simulink model "Demo_V2X_RoadWorks_cs"  (R2014b)
settings: Solver=ode5  SolverMode=SingleTasking  StartTime=0.0  StopTime=18  FixedStep=1/100  RelTol=1e-3
PreLoadFcn:
  | mbxruntime.callbacks.PreLoadFcn(bdroot);
  | check_NUTS_defined;
  | 
  | assignin('base',['model_closed_' bdroot],false);
PostLoadFcn:
  | mbxruntime.callbacks.PostLoadFcn(bdroot);
InitFcn:
  | mbxruntime.callbacks.InitFcn(bdroot);
StartFcn:
  | mbxruntime.callbacks.StartFcn(bdroot);
StopFcn:
  | mbxruntime.callbacks.StopFcn(bdroot);
model workspace: external: MAT-File .\Demo_V2X_RoadWorks_cs_hws.mat (data not in the file)
undefined symbols (not defined in the file or in its folder): InitializeBus, mbxruntime, Newton, Raphson, tabledata
undefined symbols (not defined in the file): Demo_V2X_RoadWorks_cs_002408181c311178, Demo_V2X_RoadWorks_cs_02afd40c5576fd79, Demo_V2X_RoadWorks_cs_09062d95c4976b80, Demo_V2X_RoadWorks_cs_0ad60e46608f1bfe, Demo_V2X_RoadWorks_cs_0b386a01b2cd5e8d, Demo_V2X_RoadWorks_cs_0d795afaa024d2ee, Demo_V2X_RoadWorks_cs_104085e65c337077, Demo_V2X_RoadWorks_cs_126564f7b2997a49, Demo_V2X_RoadWorks_cs_15e6e2595e8bf329, Demo_V2X_RoadWorks_cs_16adfea7655bce18, Demo_V2X_RoadWorks_cs_18ab2686f8449f50, Demo_V2X_RoadWorks_cs_1c28437def32f9f6, Demo_V2X_RoadWorks_cs_1d541c73c3d8f25b, Demo_V2X_RoadWorks_cs_1fb1f994fe012d27, Demo_V2X_RoadWorks_cs_20c117b9827230b9, Demo_V2X_RoadWorks_cs_220b1226a84e3b37, Demo_V2X_RoadWorks_cs_24814049c8ab2e18, Demo_V2X_RoadWorks_cs_24a281220a6492a7, Demo_V2X_RoadWorks_cs_279aea126b4236ad, Demo_V2X_RoadWorks_cs_28eadd0b23e572db, Demo_V2X_RoadWorks_cs_291fe7210f9ba434, Demo_V2X_RoadWorks_cs_2fd90504f8814746, Demo_V2X_RoadWorks_cs_33c1737bfc1c651f, Demo_V2X_RoadWorks_cs_388e22d5b1056b8f, Demo_V2X_RoadWorks_cs_3e3a415e868663e7, Demo_V2X_RoadWorks_cs_45759eb0c1816b1e, Demo_V2X_RoadWorks_cs_45f301cf6c396570, Demo_V2X_RoadWorks_cs_47686124f5151dea, Demo_V2X_RoadWorks_cs_487931e8a8cef1d6, Demo_V2X_RoadWorks_cs_54cb5626dca53ab7, Demo_V2X_RoadWorks_cs_56c0a253fe7e7ec0, Demo_V2X_RoadWorks_cs_5921488c0ba4168e, Demo_V2X_RoadWorks_cs_5ca0c70551eea1b3, Demo_V2X_RoadWorks_cs_5cc6ddb60eb17926, Demo_V2X_RoadWorks_cs_5dda33a127b53dd9, Demo_V2X_RoadWorks_cs_60729aca19e3b8ea, Demo_V2X_RoadWorks_cs_61616eaaf58ec115, Demo_V2X_RoadWorks_cs_63af626c9fae5224, Demo_V2X_RoadWorks_cs_649c6af7b111a61f, Demo_V2X_RoadWorks_cs_64e2df335ac415c1, Demo_V2X_RoadWorks_cs_6530f1ae727e39fe, Demo_V2X_RoadWorks_cs_6837be8d052ff1e3, Demo_V2X_RoadWorks_cs_6e8b51a123f1a201, Demo_V2X_RoadWorks_cs_6f4ec518a68cacb3, Demo_V2X_RoadWorks_cs_74dac4a6b9859226, Demo_V2X_RoadWorks_cs_75671d8cae67d5b6, Demo_V2X_RoadWorks_cs_756d40a88ae84d39, Demo_V2X_RoadWorks_cs_77c7cbc4fa1cdaa5, Demo_V2X_RoadWorks_cs_7b9fbc44403bb8f3, Demo_V2X_RoadWorks_cs_7c118b74c8d14c00, Demo_V2X_RoadWorks_cs_7c4a172761f05beb, Demo_V2X_RoadWorks_cs_80b7a78efe24d5f1, Demo_V2X_RoadWorks_cs_82d65efce1f7c4ea, Demo_V2X_RoadWorks_cs_8be5dc2565229ce9, Demo_V2X_RoadWorks_cs_8dc36f0ab6cec640, Demo_V2X_RoadWorks_cs_91305dd1362bb00d, Demo_V2X_RoadWorks_cs_929c2ffed1faf33f, Demo_V2X_RoadWorks_cs_95615bcbc0d062f1, Demo_V2X_RoadWorks_cs_99a6391a40f894df, Demo_V2X_RoadWorks_cs_9caa19175765ea5d ... (+52)
libraries: PreScanSimulinkLibrary x34, simulink_extras x15, simulink x6
(part 16 of 16)

== matlab function Demo_V2X_RoadWorks_cs/Actros_2541_1/V2X_6201_DENM_Create ==
  data: PRESCAN_V2X_FIXED_DENM_MESSAGE_zero_init parameter Bus: PRESCAN_V2X_FIXED_DENM_MESSAGE; message output Bus: PRESCAN_V2X_FIXED_DENM_MESSAGE; z input
function message = update(PRESCAN_V2X_FIXED_DENM_MESSAGE_zero_init, z)
%#codegen

message = PRESCAN_V2X_FIXED_DENM_MESSAGE_zero_init;
message.HEADER.valid = true;

% The lines below are example assignments that can be uncommented
% and changed as needed to construct a message to be sent.

% message.DATA.header.protocolVersion = int32(1);
% message.DATA.header.messageID = int32(1);
% message.DATA.header.stationID = int32(1);
% message.DATA.denm.management.actionID.originatingStationID = int32(1);
% message.DATA.denm.management.actionID.sequenceNumber = int32(1);
% message.DATA.denm.management.eventPosition.positionConfidenceEllipse.semiMajorConfidence = int32(1);
% message.DATA.denm.management.eventPosition.positionConfidenceEllipse.semiMinorConfidence = int32(1);
% message.DATA.denm.management.eventPosition.positionConfidenceEllipse.semiMajorOrientation = int32(1);
% message.DATA.denm.management.eventPosition.altitude.altitudeValue = int32(1);
% message.DATA.denm.management.eventPosition.altitude.altitudeConfidence = int32(1);
% message.DATA.denm.management.eventPosition.latitude = int32(1);
% message.DATA.denm.management.eventPosition.longitude = int32(1);
% message.DATA.denm.management.detectionTime = int32(1);
% message.DATA.denm.management.referenceTime = int32(1);
% message.DATA.denm.management.termination = int32(1);
% message.DATA.denm.management.relevanceDistance = int32(1);
% message.DATA.denm.management.relevanceTrafficDirection = int32(1);
% message.DATA.denm.management.validityDuration = int32(1);
% message.DATA.denm.management.transmissionInterval = int32(1);
% message.DATA.denm.management.stationType = int32(1);
% message.DATA.denm.situation.eventType.causeCode = int32(1);
% message.DATA.denm.situation.eventType.subCauseCode = int32(1);
% message.DATA.denm.situation.linkedCause.causeCode = int32(1);
% message.DATA.denm.situation.linkedCause.subCauseCode = int32(1);
% message.DATA.denm.situation.eventHistory(1).eventPosition.deltaLatitude = int32(1);
% message.DATA.denm.situation.eventHistory(1).eventPosition.deltaLongitude = int32(1);
% message.DATA.denm.situation.eventHistory(1).eventPosition.deltaAltitude = int32(1);
% message.DATA.denm.situation.eventHistory(1).eventDeltaTime = int32(1);
% message.DATA.denm.situation.eventHistory(1).informationQuality = int32(1);
% message.DATA.denm.situation.informationQuality = int32(1);
% % message.DATA.denm.situation.eventHistory(1) is an array
% message.DATA.denm.location.eventSpeed.speedValue = int32(1);
% message.DATA.denm.location.eventSpeed.speedConfidence = int32(1);
% message.DATA.denm.location.eventPositionHeading.headingValue = int32(1);
% message.DATA.denm.location.eventPositionHeading.headingConfidence = int32(1);
% message.DATA.denm.location.traces(1).pathPosition.deltaLatitude = int32(1);
% message.DATA.denm.location.traces(1).pathPosition.deltaLongitude = int32(1);
% message.DATA.denm.location.traces(1).pathPosition.deltaAltitude = int32(1);
% message.DATA.denm.location.traces(1).pathDeltaTime = int32(1);
% % message.DATA.denm.location.traces(1) is an array
% message.DATA.denm.location.roadType = int32(1);
% message.DATA.denm.alacarte.impactReduction.heightLonCarrLeft = int32(1);
% message.DATA.denm.alacarte.impactReduction.heightLonCarrRight = int32(1);
% message.DATA.denm.alacarte.impactReduction.posLonCarrLeft = int32(1);
% message.DATA.denm.alacarte.impactReduction.posLonCarrRight = int32(1);
% % message.DATA.denm.alacarte.impactReduction.positionOfPillars(1) is an array
% message.DATA.denm.alacarte.impactReduction.posCentMass = int32(1);
% message.DATA.denm.alacarte.impactReduction.wheelBaseVehicle = int32(1);
% message.DATA.denm.alacarte.impactReduction.turningRadius = int32(1);
% message.DATA.denm.alacarte.impactReduction.posFrontAx = int32(1);
% message.DATA.denm.alacarte.impactReduction.positionOfOccupants = int32(1);
% message.DATA.denm.alacarte.impactReduction.vehicleMass = int32(1);
% message.DATA.denm.alacarte.impactReduction.requestResponseIndication = int32(1);
% message.DATA.denm.alacarte.roadWorks.closedLanes.hardShoulderStatus = int32(1);
% message.DATA.denm.alacarte.roadWorks.closedLanes.drivingLaneStatus = int32(1);
% message.DATA.denm.alacarte.roadWorks.incidentIndication.causeCode = int32(1);
% message.DATA.denm.alacarte.roadWorks.incidentIndication.subCauseCode = int32(1);
% message.DATA.denm.alacarte.roadWorks.recommendedPath(1).positionConfidenceEllipse.semiMajorConfidence = int32(1);
% message.DATA.denm.alacarte.roadWorks.recommendedPath(1).positionConfidenceEllipse.semiMinorConfidence = int32(1);
% message.DATA.denm.alacarte.roadWorks.recommendedPath(1).positionConfidenceEllipse.semiMajorOrientation = int32(1);
% message.DATA.denm.alacarte.roadWorks.recommendedPath(1).altitude.altitudeValue = int32(1);
% message.DATA.denm.alacarte.roadWorks.recommendedPath(1).altitude.altitudeConfidence = int32(1);
% message.DATA.denm.alacarte.roadWorks.recommendedPath(1).latitude = int32(1);
% message.DATA.denm.alacarte.roadWorks.recommendedPath(1).longitude = int32(1);
% message.DATA.denm.alacarte.roadWorks.startingPointSpeedLimit.deltaLatitude = int32(1);
% message.DATA.denm.alacarte.roadWorks.startingPointSpeedLimit.deltaLongitude = int32(1);
% message.DATA.denm.alacarte.roadWorks.startingPointSpeedLimit.deltaAltitude = int32(1);
% message.DATA.denm.alacarte.roadWorks.referenceDenms(1).originatingStationID = int32(1);
% message.DATA.denm.alacarte.roadWorks.referenceDenms(1).sequenceNumber = int32(1);
% message.DATA.denm.alacarte.roadWorks.lightBarSirenInUse = int32(1);
% % message.DATA.denm.alacarte.roadWorks.restriction(1) is an array
% message.DATA.denm.alacarte.roadWorks.speedLimit = int32(1);
% % message.DATA.denm.alacarte.roadWorks.recommendedPath(1) is an array
% message.DATA.denm.alacarte.roadWorks.trafficFlowRule = int32(1);
% % message.DATA.denm.alacarte.roadWorks.referenceDenms(1) is an array
% message.DATA.denm.alacarte.stationaryVehicle.stationaryCause.causeCode = int32(1);
% message.DATA.denm.alacarte.stationaryVehicle.stationaryCause.subCauseCode = int32(1);
% message.DATA.denm.alacarte.stationaryVehicle.carryingDangerousGoods.dangerousGoodsType = int32(1);
% message.DATA.denm.alacarte.stationaryVehicle.carryingDangerousGoods.unNumber = int32(1);
% message.DATA.denm.alacarte.stationaryVehicle.carryingDangerousGoods.elevatedTemperature = logical(1);
% message.DATA.denm.alacarte.stationaryVehicle.carryingDangerousGoods.tunnelsRestricted = logical(1);
% message.DATA.denm.alacarte.stationaryVehicle.carryingDangerousGoods.limitedQuantity = logical(1);
% message.DATA.denm.alacarte.stationaryVehicle.carryingDangerousGoods.emergencyActionCode = int8(zeros(24, 1)); % Array up to 24 bytes
% message.DATA.denm.alacarte.stationaryVehicle.carryingDangerousGoods.phoneNumber = int8(zeros(24, 1)); % Array up to 24 bytes
% message.DATA.denm.alacarte.stationaryVehicle.carryingDangerousGoods.companyName = int8(zeros(24, 1)); % Array up to 24 bytes
% message.DATA.denm.alacarte.stationaryVehicle.vehicleIdentification.wMInumber = int8(zeros(3, 1)); % Array up to 3 bytes
% message.DATA.denm.alacarte.stationaryVehicle.vehicleIdentification.vDS = int8(zeros(6, 1)); % Array up to 6 bytes
% message.DATA.denm.alacarte.stationaryVehicle.stationarySince = int32(1);
% message.DATA.denm.alacarte.stationaryVehicle.numberOfOccupants = int32(1);
% message.DATA.denm.alacarte.stationaryVehicle.energyStorageType = int32(1);
% message.DATA.denm.alacarte.lanePosition = int32(1);
% message.DATA.denm.alacarte.externalTemperature = int32(1);
% message.DATA.denm.alacarte.positioningSolution = int32(1);

== matlab function Demo_V2X_RoadWorks_cs/Actros_1860_1/V2X_6202_CAM_Create ==
  data: PRESCAN_V2X_FIXED_CAM_MESSAGE_zero_init parameter Bus: PRESCAN_V2X_FIXED_CAM_MESSAGE; message output Bus: PRESCAN_V2X_FIXED_CAM_MESSAGE; z input
function message = update(PRESCAN_V2X_FIXED_CAM_MESSAGE_zero_init, z)
%#codegen

message = PRESCAN_V2X_FIXED_CAM_MESSAGE_zero_init;
message.HEADER.valid = true;

% The lines below are example assignments that can be uncommented
% and changed as needed to construct a message to be sent.

% message.DATA.header.protocolVersion = int32(1);
% message.DATA.header.messageID = int32(1);
% message.DATA.header.stationID = int32(1);
% message.DATA.cam.camParameters.basicContainer.referencePosition.positionConfidenceEllipse.semiMajorConfidence = int32(1);
% message.DATA.cam.camParameters.basicContainer.referencePosition.positionConfidenceEllipse.semiMinorConfidence = int32(1);
% message.DATA.cam.camParameters.basicContainer.referencePosition.positionConfidenceEllipse.semiMajorOrientation = int32(1);
% message.DATA.cam.camParameters.basicContainer.referencePosition.altitude.altitudeValue = int32(1);
% message.DATA.cam.camParameters.basicContainer.referencePosition.altitude.altitudeConfidence = int32(1);
% message.DATA.cam.camParameters.basicContainer.referencePosition.latitude = int32(1);
% message.DATA.cam.camParameters.basicContainer.referencePosition.longitude = int32(1);
% message.DATA.cam.camParameters.basicContainer.stationType = int32(1);
% message.DATA.cam.camParameters.highFrequencyContainer.basicVehicleContainerHighFrequency.heading.headingValue = int32(1);
% message.DATA.cam.camParameters.highFrequencyContainer.basicVehicleContainerHighFrequency.heading.headingConfidence = int32(1);
% message.DATA.cam.camParameters.highFrequencyContainer.basicVehicleContainerHighFrequency.speed.speedValue = int32(1);
% message.DATA.cam.camParameters.highFrequencyContainer.basicVehicleContainerHighFrequency.speed.speedConfidence = int32(1);
% message.DATA.cam.camParameters.highFrequencyContainer.basicVehicleContainerHighFrequency.vehicleLength.vehicleLengthValue = int32(1);
% message.DATA.cam.camParameters.highFrequencyContainer.basicVehicleContainerHighFrequency.vehicleLength.vehicleLengthConfidenceIndication = int32(1);
% message.DATA.cam.camParameters.highFrequencyContainer.basicVehicleContainerHighFrequency.longitudinalAcceleration.longitudinalAccelerationValue = int32(1);
% message.DATA.cam.camParameters.highFrequencyContainer.basicVehicleContainerHighFrequency.longitudinalAcceleration.longitudinalAccelerationConfidence = int32(1);
% message.DATA.cam.camParameters.highFrequencyContainer.basicVehicleContainerHighFrequency.curvature.curvatureValue = int32(1);
% message.DATA.cam.camParameters.highFrequencyContainer.basicVehicleContainerHighFrequency.curvature.curvatureConfidence = int32(1);
% message.DATA.cam.camParameters.highFrequencyContainer.basicVehicleContainerHighFrequency.yawRate.yawRateValue = int32(1);
% message.DATA.cam.camParameters.highFrequencyContainer.basicVehicleContainerHighFrequency.yawRate.yawRateConfidence = int32(1);
% message.DATA.cam.camParameters.highFrequencyContainer.basicVehicleContainerHighFrequency.steeringWheelAngle.steeringWheelAngleValue = int32(1);
% message.DATA.cam.camParameters.highFrequencyContainer.basicVehicleContainerHighFrequency.steeringWheelAngle.steeringWheelAngleConfidence = int32(1);
% message.DATA.cam.camParameters.highFrequencyContainer.basicVehicleContainerHighFrequency.lateralAcceleration.lateralAccelerationValue = int32(1);
% message.DATA.cam.camParameters.highFrequencyContainer.basicVehicleContainerHighFrequency.lateralAcceleration.lateralAccelerationConfidence = int32(1);
% message.DATA.cam.camParameters.highFrequencyContainer.basicVehicleContainerHighFrequency.verticalAcceleration.verticalAccelerationValue = int32(1);
% message.DATA.cam.camParameters.highFrequencyContainer.basicVehicleContainerHighFrequency.verticalAcceleration.verticalAccelerationConfidence = int32(1);
% message.DATA.cam.camParameters.highFrequencyContainer.basicVehicleContainerHighFrequency.cenDsrcTollingZone.protectedZoneLatitude = int32(1);
% message.DATA.cam.camParameters.highFrequencyContainer.basicVehicleContainerHighFrequency.cenDsrcTollingZone.protectedZoneLongitude = int32(1);
% message.DATA.cam.camParameters.highFrequencyContainer.basicVehicleContainerHighFrequency.cenDsrcTollingZone.cenDsrcTollingZoneID = int32(1);
% message.DATA.cam.camParameters.highFrequencyContainer.basicVehicleContainerHighFrequency.driveDirection = int32(1);
% message.DATA.cam.camParameters.highFrequencyContainer.basicVehicleContainerHighFrequency.vehicleWidth = int32(1);
% message.DATA.cam.camParameters.highFrequencyContainer.basicVehicleContainerHighFrequency.curvatureCalculationMode = int32(1);
% message.DATA.cam.camParameters.highFrequencyContainer.basicVehicleContainerHighFrequency.accelerationControl = int32(1);
% message.DATA.cam.camParameters.highFrequencyContainer.basicVehicleContainerHighFrequency.lanePosition = int32(1);
% message.DATA.cam.camParameters.highFrequencyContainer.basicVehicleContainerHighFrequency.performanceClass = int32(1);
% message.DATA.cam.camParameters.highFrequencyContainer.rsuContainerHighFrequency.protectedCommunicationZonesRSU(1).protectedZoneType = int32(1);
% message.DATA.cam.camParameters.highFrequencyContainer.rsuContainerHighFrequency.protectedCommunicationZonesRSU(1).expiryTime = int32(1);
% message.DATA.cam.camParameters.highFrequencyContainer.rsuContainerHighFrequency.protectedCommunicationZonesRSU(1).protectedZoneLatitude = int32(1);
% message.DATA.cam.camParameters.highFrequencyContainer.rsuContainerHighFrequency.protectedCommunicationZonesRSU(1).protectedZoneLongitude = int32(1);
% message.DATA.cam.camParameters.highFrequencyContainer.rsuContainerHighFrequency.protectedCommunicationZonesRSU(1).protectedZoneRadius = int32(1);
% message.DATA.cam.camParameters.highFrequencyContainer.rsuContainerHighFrequency.protectedCommunicationZonesRSU(1).protectedZoneID = int32(1);
% % message.DATA.cam.camParameters.highFrequencyContainer.rsuContainerHighFrequency.protectedCommunicationZonesRSU(1) is an array
% message.DATA.cam.camParameters.lowFrequencyContainer.basicVehicleContainerLowFrequency.pathHistory(1).pathPosition.deltaLatitude = int32(1);
% message.DATA.cam.camParameters.lowFrequencyContainer.basicVehicleContainerLowFrequency.pathHistory(1).pathPosition.deltaLongitude = int32(1);
% message.DATA.cam.camParameters.lowFrequencyContainer.basicVehicleContainerLowFrequency.pathHistory(1).pathPosition.deltaAltitude = int32(1);
% message.DATA.cam.camParameters.lowFrequencyContainer.basicVehicleContainerLowFrequency.pathHistory(1).pathDeltaTime = int32(1);
% message.DATA.cam.camParameters.lowFrequencyContainer.basicVehicleContainerLowFrequency.vehicleRole = int32(1);
% message.DATA.cam.camParameters.lowFrequencyContainer.basicVehicleContainerLowFrequency.exteriorLights = int32(1);
% % message.DATA.cam.camParameters.lowFrequencyContainer.basicVehicleContainerLowFrequency.pathHistory(1) is an array
% message.DATA.cam.camParameters.specialVehicleContainer.publicTransportContainer.ptActivation.ptActivationType = int32(1);
% message.DATA.cam.camParameters.specialVehicleContainer.publicTransportContainer.ptActivation.ptActivationData = int8(zeros(20, 1)); % Array up to 20 bytes
% message.DATA.cam.camParameters.specialVehicleContainer.publicTransportContainer.embarkationStatus = logical(1);
% message.DATA.cam.camParameters.specialVehicleContainer.specialTransportContainer.specialTransportType = int32(1);
% message.DATA.cam.camParameters.specialVehicleContainer.specialTransportContainer.lightBarSirenInUse = int32(1);
% message.DATA.cam.camParameters.specialVehicleContainer.dangerousGoodsContainer.dangerousGoodsBasic = int32(1);
% message.DATA.cam.camParameters.specialVehicleContainer.roadWorksContainerBasic.closedLanes.hardShoulderStatus = int32(1);
% message.DATA.cam.camParameters.specialVehicleContainer.roadWorksContainerBasic.closedLanes.drivingLaneStatus = int32(1);
% message.DATA.cam.camParameters.specialVehicleContainer.roadWorksContainerBasic.roadworksSubCauseCode = int32(1);
% message.DATA.cam.camParameters.specialVehicleContainer.roadWorksContainerBasic.lightBarSirenInUse = int32(1);
% message.DATA.cam.camParameters.specialVehicleContainer.rescueContainer.lightBarSirenInUse = int32(1);
% message.DATA.cam.camParameters.specialVehicleContainer.emergencyContainer.incidentIndication.causeCode = int32(1);
% message.DATA.cam.camParameters.specialVehicleContainer.emergencyContainer.incidentIndication.subCauseCode = int32(1);
% message.DATA.cam.camParameters.specialVehicleContainer.emergencyContainer.lightBarSirenInUse = int32(1);
% message.DATA.cam.camParameters.specialVehicleContainer.emergencyContainer.emergencyPriority = int32(1);
% message.DATA.cam.camParameters.specialVehicleContainer.safetyCarContainer.incidentIndication.causeCode = int32(1);
% message.DATA.cam.camParameters.specialVehicleContainer.safetyCarContainer.incidentIndication.subCauseCode = int32(1);
% message.DATA.cam.camParameters.specialVehicleContainer.safetyCarContainer.lightBarSirenInUse = int32(1);
% message.DATA.cam.camParameters.specialVehicleContainer.safetyCarContainer.trafficRule = int32(1);
% message.DATA.cam.camParameters.specialVehicleContainer.safetyCarContainer.speedLimit = int32(1);
% message.DATA.cam.generationDeltaTime = int32(1);

== matlab function Demo_V2X_RoadWorks_cs/Actros_1860_1/V2X_6202_DENM_Create ==
  data: PRESCAN_V2X_FIXED_DENM_MESSAGE_zero_init parameter Bus: PRESCAN_V2X_FIXED_DENM_MESSAGE; message output Bus: PRESCAN_V2X_FIXED_DENM_MESSAGE; z input
function message = update(PRESCAN_V2X_FIXED_DENM_MESSAGE_zero_init, z)
%#codegen

message = PRESCAN_V2X_FIXED_DENM_MESSAGE_zero_init;
message.HEADER.valid = true;

% The lines below are example assignments that can be uncommented
% and changed as needed to construct a message to be sent.

% message.DATA.header.protocolVersion = int32(1);
% message.DATA.header.messageID = int32(1);
% message.DATA.header.stationID = int32(1);
% message.DATA.denm.management.actionID.originatingStationID = int32(1);
% message.DATA.denm.management.actionID.sequenceNumber = int32(1);
% message.DATA.denm.management.eventPosition.positionConfidenceEllipse.semiMajorConfidence = int32(1);
% message.DATA.denm.management.eventPosition.positionConfidenceEllipse.semiMinorConfidence = int32(1);
% message.DATA.denm.management.eventPosition.positionConfidenceEllipse.semiMajorOrientation = int32(1);
% message.DATA.denm.management.eventPosition.altitude.altitudeValue = int32(1);
% message.DATA.denm.management.eventPosition.altitude.altitudeConfidence = int32(1);
% message.DATA.denm.management.eventPosition.latitude = int32(1);
% message.DATA.denm.management.eventPosition.longitude = int32(1);
% message.DATA.denm.management.detectionTime = int32(1);
% message.DATA.denm.management.referenceTime = int32(1);
% message.DATA.denm.management.termination = int32(1);
% message.DATA.denm.management.relevanceDistance = int32(1);
% message.DATA.denm.management.relevanceTrafficDirection = int32(1);
% message.DATA.denm.management.validityDuration = int32(1);
% message.DATA.denm.management.transmissionInterval = int32(1);
% message.DATA.denm.management.stationType = int32(1);
% message.DATA.denm.situation.eventType.causeCode = int32(1);
% message.DATA.denm.situation.eventType.subCauseCode = int32(1);
% message.DATA.denm.situation.linkedCause.causeCode = int32(1);
% message.DATA.denm.situation.linkedCause.subCauseCode = int32(1);
% message.DATA.denm.situation.eventHistory(1).eventPosition.deltaLatitude = int32(1);
% message.DATA.denm.situation.eventHistory(1).eventPosition.deltaLongitude = int32(1);
% message.DATA.denm.situation.eventHistory(1).eventPosition.deltaAltitude = int32(1);
% message.DATA.denm.situation.eventHistory(1).eventDeltaTime = int32(1);
% message.DATA.denm.situation.eventHistory(1).informationQuality = int32(1);
% message.DATA.denm.situation.informationQuality = int32(1);
% % message.DATA.denm.situation.eventHistory(1) is an array
% message.DATA.denm.location.eventSpeed.speedValue = int32(1);
% message.DATA.denm.location.eventSpeed.speedConfidence = int32(1);
% message.DATA.denm.location.eventPositionHeading.headingValue = int32(1);
% message.DATA.denm.location.eventPositionHeading.headingConfidence = int32(1);
% message.DATA.denm.location.traces(1).pathPosition.deltaLatitude = int32(1);
% message.DATA.denm.location.traces(1).pathPosition.deltaLongitude = int32(1);
% message.DATA.denm.location.traces(1).pathPosition.deltaAltitude = int32(1);
% message.DATA.denm.location.traces(1).pathDeltaTime = int32(1);
% % message.DATA.denm.location.traces(1) is an array
% message.DATA.denm.location.roadType = int32(1);
% message.DATA.denm.alacarte.impactReduction.heightLonCarrLeft = int32(1);
% message.DATA.denm.alacarte.impactReduction.heightLonCarrRight = int32(1);
% message.DATA.denm.alacarte.impactReduction.posLonCarrLeft = int32(1);
% message.DATA.denm.alacarte.impactReduction.posLonCarrRight = int32(1);
% % message.DATA.denm.alacarte.impactReduction.positionOfPillars(1) is an array
% message.DATA.denm.alacarte.impactReduction.posCentMass = int32(1);
% message.DATA.denm.alacarte.impactReduction.wheelBaseVehicle = int32(1);
% message.DATA.denm.alacarte.impactReduction.turningRadius = int32(1);
% message.DATA.denm.alacarte.impactReduction.posFrontAx = int32(1);
% message.DATA.denm.alacarte.impactReduction.positionOfOccupants = int32(1);
% message.DATA.denm.alacarte.impactReduction.vehicleMass = int32(1);
% message.DATA.denm.alacarte.impactReduction.requestResponseIndication = int32(1);
% message.DATA.denm.alacarte.roadWorks.closedLanes.hardShoulderStatus = int32(1);
% message.DATA.denm.alacarte.roadWorks.closedLanes.drivingLaneStatus = int32(1);
% message.DATA.denm.alacarte.roadWorks.incidentIndication.causeCode = int32(1);
% message.DATA.denm.alacarte.roadWorks.incidentIndication.subCauseCode = int32(1);
% message.DATA.denm.alacarte.roadWorks.recommendedPath(1).positionConfidenceEllipse.semiMajorConfidence = int32(1);
% message.DATA.denm.alacarte.roadWorks.recommendedPath(1).positionConfidenceEllipse.semiMinorConfidence = int32(1);
% message.DATA.denm.alacarte.roadWorks.recommendedPath(1).positionConfidenceEllipse.semiMajorOrientation = int32(1);
% message.DATA.denm.alacarte.roadWorks.recommendedPath(1).altitude.altitudeValue = int32(1);
% message.DATA.denm.alacarte.roadWorks.recommendedPath(1).altitude.altitudeConfidence = int32(1);
% message.DATA.denm.alacarte.roadWorks.recommendedPath(1).latitude = int32(1);
% message.DATA.denm.alacarte.roadWorks.recommendedPath(1).longitude = int32(1);
% message.DATA.denm.alacarte.roadWorks.startingPointSpeedLimit.deltaLatitude = int32(1);
% message.DATA.denm.alacarte.roadWorks.startingPointSpeedLimit.deltaLongitude = int32(1);
% message.DATA.denm.alacarte.roadWorks.startingPointSpeedLimit.deltaAltitude = int32(1);
% message.DATA.denm.alacarte.roadWorks.referenceDenms(1).originatingStationID = int32(1);
% message.DATA.denm.alacarte.roadWorks.referenceDenms(1).sequenceNumber = int32(1);
% message.DATA.denm.alacarte.roadWorks.lightBarSirenInUse = int32(1);
% % message.DATA.denm.alacarte.roadWorks.restriction(1) is an array
% message.DATA.denm.alacarte.roadWorks.speedLimit = int32(1);
% % message.DATA.denm.alacarte.roadWorks.recommendedPath(1) is an array
% message.DATA.denm.alacarte.roadWorks.trafficFlowRule = int32(1);
% % message.DATA.denm.alacarte.roadWorks.referenceDenms(1) is an array
% message.DATA.denm.alacarte.stationaryVehicle.stationaryCause.causeCode = int32(1);
% message.DATA.denm.alacarte.stationaryVehicle.stationaryCause.subCauseCode = int32(1);
% message.DATA.denm.alacarte.stationaryVehicle.carryingDangerousGoods.dangerousGoodsType = int32(1);
% message.DATA.denm.alacarte.stationaryVehicle.carryingDangerousGoods.unNumber = int32(1);
% message.DATA.denm.alacarte.stationaryVehicle.carryingDangerousGoods.elevatedTemperature = logical(1);
% message.DATA.denm.alacarte.stationaryVehicle.carryingDangerousGoods.tunnelsRestricted = logical(1);
% message.DATA.denm.alacarte.stationaryVehicle.carryingDangerousGoods.limitedQuantity = logical(1);
% message.DATA.denm.alacarte.stationaryVehicle.carryingDangerousGoods.emergencyActionCode = int8(zeros(24, 1)); % Array up to 24 bytes
% message.DATA.denm.alacarte.stationaryVehicle.carryingDangerousGoods.phoneNumber = int8(zeros(24, 1)); % Array up to 24 bytes
% message.DATA.denm.alacarte.stationaryVehicle.carryingDangerousGoods.companyName = int8(zeros(24, 1)); % Array up to 24 bytes
% message.DATA.denm.alacarte.stationaryVehicle.vehicleIdentification.wMInumber = int8(zeros(3, 1)); % Array up to 3 bytes
% message.DATA.denm.alacarte.stationaryVehicle.vehicleIdentification.vDS = int8(zeros(6, 1)); % Array up to 6 bytes
% message.DATA.denm.alacarte.stationaryVehicle.stationarySince = int32(1);
% message.DATA.denm.alacarte.stationaryVehicle.numberOfOccupants = int32(1);
% message.DATA.denm.alacarte.stationaryVehicle.energyStorageType = int32(1);
% message.DATA.denm.alacarte.lanePosition = int32(1);
% message.DATA.denm.alacarte.externalTemperature = int32(1);
% message.DATA.denm.alacarte.positioningSolution = int32(1);

== matlab function Demo_V2X_RoadWorks_cs/CarTrailer_SingleAxle_1/V2X_6114_CAM_Create ==
  data: PRESCAN_V2X_FIXED_CAM_MESSAGE_zero_init parameter Bus: PRESCAN_V2X_FIXED_CAM_MESSAGE; message output Bus: PRESCAN_V2X_FIXED_CAM_MESSAGE; z input
function message = update(PRESCAN_V2X_FIXED_CAM_MESSAGE_zero_init, z)
%#codegen

message = PRESCAN_V2X_FIXED_CAM_MESSAGE_zero_init;
message.HEADER.valid = true;

% The lines below are example assignments that can be uncommented
% and changed as needed to construct a message to be sent.

% message.DATA.header.protocolVersion = int32(1);
% message.DATA.header.messageID = int32(1);
% message.DATA.header.stationID = int32(1);
% message.DATA.cam.camParameters.basicContainer.referencePosition.positionConfidenceEllipse.semiMajorConfidence = int32(1);
% message.DATA.cam.camParameters.basicContainer.referencePosition.positionConfidenceEllipse.semiMinorConfidence = int32(1);
% message.DATA.cam.camParameters.basicContainer.referencePosition.positionConfidenceEllipse.semiMajorOrientation = int32(1);
% message.DATA.cam.camParameters.basicContainer.referencePosition.altitude.altitudeValue = int32(1);
% message.DATA.cam.camParameters.basicContainer.referencePosition.altitude.altitudeConfidence = int32(1);
% message.DATA.cam.camParameters.basicContainer.referencePosition.latitude = int32(1);
% message.DATA.cam.camParameters.basicContainer.referencePosition.longitude = int32(1);
% message.DATA.cam.camParameters.basicContainer.stationType = int32(1);
% message.DATA.cam.camParameters.highFrequencyContainer.basicVehicleContainerHighFrequency.heading.headingValue = int32(1);
% message.DATA.cam.camParameters.highFrequencyContainer.basicVehicleContainerHighFrequency.heading.headingConfidence = int32(1);
% message.DATA.cam.camParameters.highFrequencyContainer.basicVehicleContainerHighFrequency.speed.speedValue = int32(1);
% message.DATA.cam.camParameters.highFrequencyContainer.basicVehicleContainerHighFrequency.speed.speedConfidence = int32(1);
% message.DATA.cam.camParameters.highFrequencyContainer.basicVehicleContainerHighFrequency.vehicleLength.vehicleLengthValue = int32(1);
% message.DATA.cam.camParameters.highFrequencyContainer.basicVehicleContainerHighFrequency.vehicleLength.vehicleLengthConfidenceIndication = int32(1);
% message.DATA.cam.camParameters.highFrequencyContainer.basicVehicleContainerHighFrequency.longitudinalAcceleration.longitudinalAccelerationValue = int32(1);
% message.DATA.cam.camParameters.highFrequencyContainer.basicVehicleContainerHighFrequency.longitudinalAcceleration.longitudinalAccelerationConfidence = int32(1);
% message.DATA.cam.camParameters.highFrequencyContainer.basicVehicleContainerHighFrequency.curvature.curvatureValue = int32(1);
% message.DATA.cam.camParameters.highFrequencyContainer.basicVehicleContainerHighFrequency.curvature.curvatureConfidence = int32(1);
% message.DATA.cam.camParameters.highFrequencyContainer.basicVehicleContainerHighFrequency.yawRate.yawRateValue = int32(1);
% message.DATA.cam.camParameters.highFrequencyContainer.basicVehicleContainerHighFrequency.yawRate.yawRateConfidence = int32(1);
% message.DATA.cam.camParameters.highFrequencyContainer.basicVehicleContainerHighFrequency.steeringWheelAngle.steeringWheelAngleValue = int32(1);
% message.DATA.cam.camParameters.highFrequencyContainer.basicVehicleContainerHighFrequency.steeringWheelAngle.steeringWheelAngleConfidence = int32(1);
% message.DATA.cam.camParameters.highFrequencyContainer.basicVehicleContainerHighFrequency.lateralAcceleration.lateralAccelerationValue = int32(1);
% message.DATA.cam.camParameters.highFrequencyContainer.basicVehicleContainerHighFrequency.lateralAcceleration.lateralAccelerationConfidence = int32(1);
% message.DATA.cam.camParameters.highFrequencyContainer.basicVehicleContainerHighFrequency.verticalAcceleration.verticalAccelerationValue = int32(1);
% message.DATA.cam.camParameters.highFrequencyContainer.basicVehicleContainerHighFrequency.verticalAcceleration.verticalAccelerationConfidence = int32(1);
% message.DATA.cam.camParameters.highFrequencyContainer.basicVehicleContainerHighFrequency.cenDsrcTollingZone.protectedZoneLatitude = int32(1);
% message.DATA.cam.camParameters.highFrequencyContainer.basicVehicleContainerHighFrequency.cenDsrcTollingZone.protectedZoneLongitude = int32(1);
% message.DATA.cam.camParameters.highFrequencyContainer.basicVehicleContainerHighFrequency.cenDsrcTollingZone.cenDsrcTollingZoneID = int32(1);
% message.DATA.cam.camParameters.highFrequencyContainer.basicVehicleContainerHighFrequency.driveDirection = int32(1);
% message.DATA.cam.camParameters.highFrequencyContainer.basicVehicleContainerHighFrequency.vehicleWidth = int32(1);
% message.DATA.cam.camParameters.highFrequencyContainer.basicVehicleContainerHighFrequency.curvatureCalculationMode = int32(1);
% message.DATA.cam.camParameters.highFrequencyContainer.basicVehicleContainerHighFrequency.accelerationControl = int32(1);
% message.DATA.cam.camParameters.highFrequencyContainer.basicVehicleContainerHighFrequency.lanePosition = int32(1);
% message.DATA.cam.camParameters.highFrequencyContainer.basicVehicleContainerHighFrequency.performanceClass = int32(1);
% message.DATA.cam.camParameters.highFrequencyContainer.rsuContainerHighFrequency.protectedCommunicationZonesRSU(1).protectedZoneType = int32(1);
% message.DATA.cam.camParameters.highFrequencyContainer.rsuContainerHighFrequency.protectedCommunicationZonesRSU(1).expiryTime = int32(1);
% message.DATA.cam.camParameters.highFrequencyContainer.rsuContainerHighFrequency.protectedCommunicationZonesRSU(1).protectedZoneLatitude = int32(1);
% message.DATA.cam.camParameters.highFrequencyContainer.rsuContainerHighFrequency.protectedCommunicationZonesRSU(1).protectedZoneLongitude = int32(1);
% message.DATA.cam.camParameters.highFrequencyContainer.rsuContainerHighFrequency.protectedCommunicationZonesRSU(1).protectedZoneRadius = int32(1);
% message.DATA.cam.camParameters.highFrequencyContainer.rsuContainerHighFrequency.protectedCommunicationZonesRSU(1).protectedZoneID = int32(1);
% % message.DATA.cam.camParameters.highFrequencyContainer.rsuContainerHighFrequency.protectedCommunicationZonesRSU(1) is an array
% message.DATA.cam.camParameters.lowFrequencyContainer.basicVehicleContainerLowFrequency.pathHistory(1).pathPosition.deltaLatitude = int32(1);
% message.DATA.cam.camParameters.lowFrequencyContainer.basicVehicleContainerLowFrequency.pathHistory(1).pathPosition.deltaLongitude = int32(1);
% message.DATA.cam.camParameters.lowFrequencyContainer.basicVehicleContainerLowFrequency.pathHistory(1).pathPosition.deltaAltitude = int32(1);
% message.DATA.cam.camParameters.lowFrequencyContainer.basicVehicleContainerLowFrequency.pathHistory(1).pathDeltaTime = int32(1);
% message.DATA.cam.camParameters.lowFrequencyContainer.basicVehicleContainerLowFrequency.vehicleRole = int32(1);
% message.DATA.cam.camParameters.lowFrequencyContainer.basicVehicleContainerLowFrequency.exteriorLights = int32(1);
% % message.DATA.cam.camParameters.lowFrequencyContainer.basicVehicleContainerLowFrequency.pathHistory(1) is an array
% message.DATA.cam.camParameters.specialVehicleContainer.publicTransportContainer.ptActivation.ptActivationType = int32(1);
% message.DATA.cam.camParameters.specialVehicleContainer.publicTransportContainer.ptActivation.ptActivationData = int8(zeros(20, 1)); % Array up to 20 bytes
% message.DATA.cam.camParameters.specialVehicleContainer.publicTransportContainer.embarkationStatus = logical(1);
% message.DATA.cam.camParameters.specialVehicleContainer.specialTransportContainer.specialTransportType = int32(1);
% message.DATA.cam.camParameters.specialVehicleContainer.specialTransportContainer.lightBarSirenInUse = int32(1);
% message.DATA.cam.camParameters.specialVehicleContainer.dangerousGoodsContainer.dangerousGoodsBasic = int32(1);
% message.DATA.cam.camParameters.specialVehicleContainer.roadWorksContainerBasic.closedLanes.hardShoulderStatus = int32(1);
% message.DATA.cam.camParameters.specialVehicleContainer.roadWorksContainerBasic.closedLanes.drivingLaneStatus = int32(1);
% message.DATA.cam.camParameters.specialVehicleContainer.roadWorksContainerBasic.roadworksSubCauseCode = int32(1);
% message.DATA.cam.camParameters.specialVehicleContainer.roadWorksContainerBasic.lightBarSirenInUse = int32(1);
% message.DATA.cam.camParameters.specialVehicleContainer.rescueContainer.lightBarSirenInUse = int32(1);
% message.DATA.cam.camParameters.specialVehicleContainer.emergencyContainer.incidentIndication.causeCode = int32(1);
% message.DATA.cam.camParameters.specialVehicleContainer.emergencyContainer.incidentIndication.subCauseCode = int32(1);
% message.DATA.cam.camParameters.specialVehicleContainer.emergencyContainer.lightBarSirenInUse = int32(1);
% message.DATA.cam.camParameters.specialVehicleContainer.emergencyContainer.emergencyPriority = int32(1);
% message.DATA.cam.camParameters.specialVehicleContainer.safetyCarContainer.incidentIndication.causeCode = int32(1);
% message.DATA.cam.camParameters.specialVehicleContainer.safetyCarContainer.incidentIndication.subCauseCode = int32(1);
% message.DATA.cam.camParameters.specialVehicleContainer.safetyCarContainer.lightBarSirenInUse = int32(1);
% message.DATA.cam.camParameters.specialVehicleContainer.safetyCarContainer.trafficRule = int32(1);
% message.DATA.cam.camParameters.specialVehicleContainer.safetyCarContainer.speedLimit = int32(1);
% message.DATA.cam.generationDeltaTime = int32(1);

== matlab function Demo_V2X_RoadWorks_cs/CarTrailer_SingleAxle_1/V2X_6114_DENM_Create ==
  data: PRESCAN_V2X_FIXED_DENM_MESSAGE_zero_init parameter Bus: PRESCAN_V2X_FIXED_DENM_MESSAGE; message output Bus: PRESCAN_V2X_FIXED_DENM_MESSAGE; stationID input; detectionTime input; gpsLatLon input; altitude input; heading input
function message = update(PRESCAN_V2X_FIXED_DENM_MESSAGE_zero_init, stationID, detectionTime, gpsLatLon, altitude, heading)
%#codegen

message = PRESCAN_V2X_FIXED_DENM_MESSAGE_zero_init;
message.HEADER.valid = true;

% The lines below are example assignments that can be uncommented
% and changed as needed to construct a message to be sent.

% message.DATA.header.protocolVersion = int32(1);
% message.DATA.header.messageID = int32(1);
message.DATA.header.stationID = stationID;
message.DATA.denm.management.actionID.originatingStationID = stationID;
% message.DATA.denm.management.actionID.sequenceNumber = int32(1);
% message.DATA.denm.management.eventPosition.positionConfidenceEllipse.semiMajorConfidence = int32(1);
% message.DATA.denm.management.eventPosition.positionConfidenceEllipse.semiMinorConfidence = int32(1);
message.DATA.denm.management.eventPosition.positionConfidenceEllipse.semiMajorOrientation = heading;
message.DATA.denm.management.eventPosition.altitude.altitudeValue = altitude;
% message.DATA.denm.management.eventPosition.altitude.altitudeConfidence = int32(1);
message.DATA.denm.management.eventPosition.latitude = gpsLatLon(1);
message.DATA.denm.management.eventPosition.longitude = gpsLatLon(2);
message.DATA.denm.management.detectionTime = detectionTime;
message.DATA.denm.management.referenceTime = detectionTime;
% message.DATA.denm.management.termination = int32(1);
message.DATA.denm.management.relevanceDistance = int32(5); % less than 5 km
message.DATA.denm.management.relevanceTrafficDirection = int32(1); % upstream_traffic
message.DATA.denm.management.validityDuration = int32(1 * 60 * 60 * 24); % 1 day in seconds
% message.DATA.denm.management.transmissionInterval = int32(1);
message.DATA.denm.management.stationType = int32(9); % trailer
message.DATA.denm.situation.eventType.causeCode = int32(3); % RoadWorks
message.DATA.denm.situation.eventType.subCauseCode = int32(4); % shortTermStationaryRoadworks
% message.DATA.denm.situation.linkedCause.causeCode = int32(1);
% message.DATA.denm.situation.linkedCause.subCauseCode = int32(1);
% message.DATA.denm.situation.eventHistory(1).eventPosition.deltaLatitude = int32(1);
% message.DATA.denm.situation.eventHistory(1).eventPosition.deltaLongitude = int32(1);
% message.DATA.denm.situation.eventHistory(1).eventPosition.deltaAltitude = int32(1);
% message.DATA.denm.situation.eventHistory(1).eventDeltaTime = int32(1);
% message.DATA.denm.situation.eventHistory(1).informationQuality = int32(1);
message.DATA.denm.situation.informationQuality = int32(7); % high
% % message.DATA.denm.situation.eventHistory(1) is an array
% message.DATA.denm.location.eventSpeed.speedValue = int32(1);
% message.DATA.denm.location.eventSpeed.speedConfidence = int32(1);
% message.DATA.denm.location.eventPositionHeading.headingValue = int32(1);
% message.DATA.denm.location.eventPositionHeading.headingConfidence = int32(1);
% message.DATA.denm.location.traces(1).pathPosition.deltaLatitude = int32(1);
% message.DATA.denm.location.traces(1).pathPosition.deltaLongitude = int32(1);
% message.DATA.denm.location.traces(1).pathPosition.deltaAltitude = int32(1);
% message.DATA.denm.location.traces(1).pathDeltaTime = int32(1);
% % message.DATA.denm.location.traces(1) is an array
% message.DATA.denm.location.roadType = int32(1);
% message.DATA.denm.alacarte.impactReduction.heightLonCarrLeft = int32(1);
% message.DATA.denm.alacarte.impactReduction.heightLonCarrRight = int32(1);
% message.DATA.denm.alacarte.impactReduction.posLonCarrLeft = int32(1);
% message.DATA.denm.alacarte.impactReduction.posLonCarrRight = int32(1);
% % message.DATA.denm.alacarte.impactReduction.positionOfPillars(1) is an array
% message.DATA.denm.alacarte.impactReduction.posCentMass = int32(1);
% message.DATA.denm.alacarte.impactReduction.wheelBaseVehicle = int32(1);
% message.DATA.denm.alacarte.impactReduction.turningRadius = int32(1);
% message.DATA.denm.alacarte.impactReduction.posFrontAx = int32(1);
% message.DATA.denm.alacarte.impactReduction.positionOfOccupants = int32(1);
% message.DATA.denm.alacarte.impactReduction.vehicleMass = int32(1);
% message.DATA.denm.alacarte.impactReduction.requestResponseIndication = int32(1);
% message.DATA.denm.alacarte.roadWorks.closedLanes.hardShoulderStatus = int32(1);
message.DATA.denm.alacarte.roadWorks.closedLanes.drivingLaneStatus = int32(1); % outerMostLaneClosed
% message.DATA.denm.alacarte.roadWorks.incidentIndication.causeCode = int32(1);
% message.DATA.denm.alacarte.roadWorks.incidentIndication.subCauseCode = int32(1);
% message.DATA.denm.alacarte.roadWorks.recommendedPath(1).positionConfidenceEllipse.semiMajorConfidence = int32(1);
% message.DATA.denm.alacarte.roadWorks.recommendedPath(1).positionConfidenceEllipse.semiMinorConfidence = int32(1);
% message.DATA.denm.alacarte.roadWorks.recommendedPath(1).positionConfidenceEllipse.semiMajorOrientation = int32(1);
% message.DATA.denm.alacarte.roadWorks.recommendedPath(1).altitude.altitudeValue = int32(1);
% message.DATA.denm.alacarte.roadWorks.recommendedPath(1).altitude.altitudeConfidence = int32(1);
% message.DATA.denm.alacarte.roadWorks.recommendedPath(1).latitude = int32(1);
% message.DATA.denm.alacarte.roadWorks.recommendedPath(1).longitude = int32(1);
% message.DATA.denm.alacarte.roadWorks.startingPointSpeedLimit.deltaLatitude = int32(1);
% message.DATA.denm.alacarte.roadWorks.startingPointSpeedLimit.deltaLongitude = int32(1);
% message.DATA.denm.alacarte.roadWorks.startingPointSpeedLimit.deltaAltitude = int32(1);
% message.DATA.denm.alacarte.roadWorks.referenceDenms(1).originatingStationID = int32(1);
% message.DATA.denm.alacarte.roadWorks.referenceDenms(1).sequenceNumber = int32(1);
% message.DATA.denm.alacarte.roadWorks.lightBarSirenInUse = int32(1);
% % message.DATA.denm.alacarte.roadWorks.restriction(1) is an array
message.DATA.denm.alacarte.roadWorks.speedLimit = int32(60); % km/H
% % message.DATA.denm.alacarte.roadWorks.recommendedPath(1) is an array
% message.DATA.denm.alacarte.roadWorks.trafficFlowRule = int32(1);
% % message.DATA.denm.alacarte.roadWorks.referenceDenms(1) is an array
% message.DATA.denm.alacarte.stationaryVehicle.stationaryCause.causeCode = int32(1);
% message.DATA.denm.alacarte.stationaryVehicle.stationaryCause.subCauseCode = int32(1);
% message.DATA.denm.alacarte.stationaryVehicle.carryingDangerousGoods.dangerousGoodsType = int32(1);
% message.DATA.denm.alacarte.stationaryVehicle.carryingDangerousGoods.unNumber = int32(1);
% message.DATA.denm.alacarte.stationaryVehicle.carryingDangerousGoods.elevatedTemperature = logical(1);
% message.DATA.denm.alacarte.stationaryVehicle.carryingDangerousGoods.tunnelsRestricted = logical(1);
% message.DATA.denm.alacarte.stationaryVehicle.carryingDangerousGoods.limitedQuantity = logical(1);
% message.DATA.denm.alacarte.stationaryVehicle.carryingDangerousGoods.emergencyActionCode = int8(zeros(24, 1)); % Array up to 24 bytes
% message.DATA.denm.alacarte.stationaryVehicle.carryingDangerousGoods.phoneNumber = int8(zeros(24, 1)); % Array up to 24 bytes
% message.DATA.denm.alacarte.stationaryVehicle.carryingDangerousGoods.companyName = int8(zeros(24, 1)); % Array up to 24 bytes
% message.DATA.denm.alacarte.stationaryVehicle.vehicleIdentification.wMInumber = int8(zeros(3, 1)); % Array up to 3 bytes
% message.DATA.denm.alacarte.stationaryVehicle.vehicleIdentification.vDS = int8(zeros(6, 1)); % Array up to 6 bytes
% message.DATA.denm.alacarte.stationaryVehicle.stationarySince = int32(1);
% message.DATA.denm.alacarte.stationaryVehicle.numberOfOccupants = int32(1);
% message.DATA.denm.alacarte.stationaryVehicle.energyStorageType = int32(1);
% message.DATA.denm.alacarte.lanePosition = int32(1);
% message.DATA.denm.alacarte.externalTemperature = int32(1);
% message.DATA.denm.alacarte.positioningSolution = int32(1);

== matlab function Demo_V2X_RoadWorks_cs/Audi_A8_1/Embedded MATLAB Function ==
  data: inbus input; outbus output Bus: PRESCAN_V2X_FIXED_DENM_MESSAGE size=1; ID input int32
function outbus  = fcn(inbus,ID)
%#eml

%initialize loop variables
k = int32(1);
outbus = inbus(1);
outbus.HEADER.valid = false;

%set the value of outbus according to the required stationID
for k = 1:length(inbus)
    if inbus(k).HEADER.valid
        stationID = inbus(k).DATA.header.stationID;
        if stationID == ID
            outbus = inbus(k);
        end
    end
end

== matlab function Demo_V2X_RoadWorks_cs/Audi_A8_1/relevantDistance Format Conversion ==
  data: relevanceDistance_m output int16; relevanceDistance input
function relevanceDistance_m = Distance_Interpretation(relevanceDistance)

switch relevanceDistance
    case 0
        relevanceDistance_m = int16(50);
    case 1
        relevanceDistance_m = int16(100);
    case 2
        relevanceDistance_m = int16(200);
    case 3
        relevanceDistance_m = int16(500);
    case 4
        relevanceDistance_m = int16(1000);
    case 5
        relevanceDistance_m = int16(5000);
    case 6
        relevanceDistance_m = int16(10000);
    otherwise
        relevanceDistance_m = int16(100000); %greater than 10km
end

== matlab function Demo_V2X_RoadWorks_cs/CarTrailer_SingleAxle_1/Date//Time Format Conversion ==
  data: Generation_Time_Epoch output
function Generation_Time_Epoch = Epoch_Time()

eml.extrinsic('now','datenum');

%Pre-allocate variables
Generation_Time = 0;
Reference_Time = 0;
Generation_Time_E = 0;

%Date/Time conversion
Generation_Time=datenum(now);                                     %Timezone - GMT+2
Reference_Time=datenum('20040101 020000.000','yyyymmdd HHMMSS');  %Reference Date/Time for the CAM/DENM - GMT/UTC
Generation_Time_E=round((Generation_Time-Reference_Time)*86400);  %Round to fix truncation

%Leap Seconds since 2004
Generation_Time_E = Generation_Time_E + 4;

Generation_Time_Epoch = int32(Generation_Time_E);
